simulink model "movePosEmg_example"  (R2017b)
settings: Solver=ode1  StartTime=0.0  StopTime=inf  FixedStep=.0005  RelTol=1e-3  EnableMultiTasking=on
libraries: CP_library x1, QB_pacer_lib x1, qbmove_library x1, simulink x1
settings Model: Creator=laurentio  LastModifiedBy=MattiaCP
settings DataIOCC: LimitDataPoints=on  SaveFormat=Array
settings OptimizationCC: LifeSpan=inf
settings DebuggingCC: UnderspecifiedInitializationDetection=Classic  MergeDetectMultiDrivingBlocksExec=none  SolverPrmCheckMsg=warning  AllowSymbolicDim=off  StateNameClashWarn=warning  SFUnexpectedBacktrackingDiag=warning  SFNoUnconditionalDefaultTransitionDiag=warning  SFExecutionAtInitializationDiag=none
settings HardwareCC: ProdBitPerPointer=32  ProdBitPerSizeT=32  ProdBitPerPtrDiffT=32  ProdLargestAtomicFloat=None  ProdIntDivRoundTo=Undefined  ProdEndianess=Unspecified  ProdWordSize=32  ProdHWDeviceType=32-bit Generic
settings ModelReferenceCC: PropagateSignalLabelsOutOfModel=off
settings CodeAppCC: StateflowObjectComments=on
settings GRTTargetCC: TargetLangStandard=C89/C90 (ANSI)  GeneratePreprocessorConditionals=Disable all
settings ConfigComp: CovMetricSettings=dw  CovHtmlReporting=on  CovSaveCumulativeToWorkspaceVar=on  CovSaveSingleToWorkspaceVar=on  CovExternalEMLEnable=off  CovSFcnEnable=off

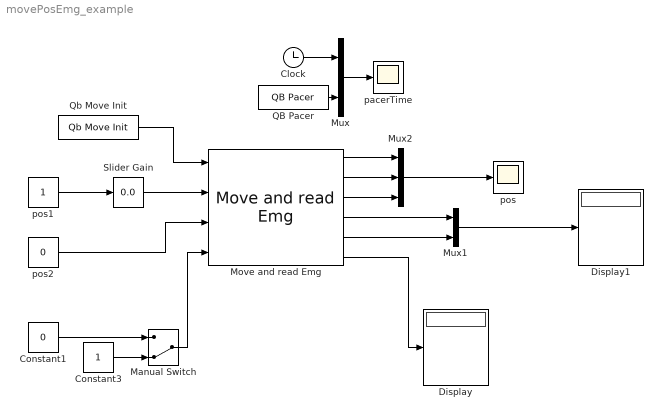
== system movePosEmg_example ==
  Clock : Clock
  Constant1 : Constant  Value=0
  Constant3 : Constant
  Display : Display
  Display1 : Display
  Manual Switch : ManualSwitch  CurrentSetting=0
  Move and read Emg : CP_library/Move and read Emg  ID=1  ACTIVE_COMM_DIRECTIONS=Both  CONTROL_MODE=Prime Movers Positions  DAISY_CHAINING=off  MAX_ANG=0  SW_LIMIT=inf  OFFSET=0  ACTIVATE=off  WDT=0  UNIT=TICK
  Mux : Mux  Inputs=2
  Mux1 : Mux  Inputs=2
  Mux2 : Mux  Inputs=3
  QB Pacer : QB_pacer_lib/QB Pacer  simTimePerRealTime=1
  Qb Move Init : qbmove_library/Qb Move Init  NUMBER_OF_COM='COM1'  BAUD_RATE_COM=2000000
      settings: SourceProductName=Qb Move Library
  Slider Gain : simulink/Math Operations/Slider Gain  gain=0.0  low=0  high=19000
  pacerTime : Scope
  pos : Scope
  pos1 : Constant
  pos2 : Constant  Value=0
  wires:
  QB Pacer/1 -> Mux/2
  Clock/1 -> Mux/1
  Qb Move Init/1 -> Move and read Emg/1
  pos1/1 -> Slider Gain/1
  Constant1/1 -> Manual Switch/1
  Slider Gain/1 -> Move and read Emg/2
  Constant3/1 -> Manual Switch/2
  pos2/1 -> Move and read Emg/3
  Move and read Emg/6 -> Display/1
  Mux/1 -> pacerTime/1
  Manual Switch/1 -> Move and read Emg/4
  Mux1/1 -> Display1/1
  Move and read Emg/4 -> Mux1/1
  Move and read Emg/5 -> Mux1/2
  Move and read Emg/1 -> Mux2/1
  Move and read Emg/2 -> Mux2/2
  Move and read Emg/3 -> Mux2/3
  Mux2/1 -> pos/1
